simulink model "simerr"  (Simulink 7.3)
settings: Solver=ode45  StartTime=0.0  StopTime=10.0  RelTol=1e-3
values from neighbouring files (symbols this model uses):
  c = v(1:D)    [canon_proj.m]
undefined symbols (not defined in the file or in its folder): a, bth, by
settings Model: Creator=locomotion  LastModifiedBy=locomotion

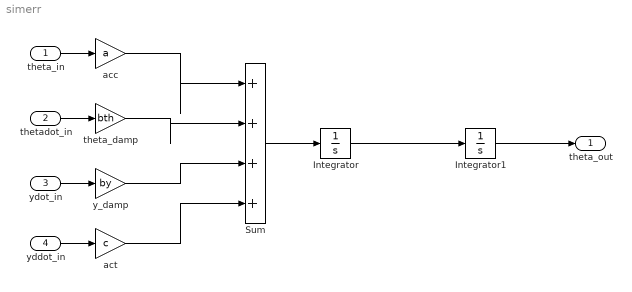
== system simerr ==
  theta_in : Inport  OutDataType=fixdt(1, 16)  OutScaling=2^0
  thetadot_in : Inport  Port=2  OutDataType=fixdt(1, 16)  OutScaling=2^0
  ydot_in : Inport  Port=3  OutDataType=fixdt(1, 16)  OutScaling=2^0
  yddot_in : Inport  Port=4  OutDataType=fixdt(1, 16)  OutScaling=2^0
  Integrator : Integrator
  Integrator1 : Integrator
  Sum : Sum  Inputs=|++++  OutDataType=fixdt(1, 16)  OutScaling=2^0
  acc : Gain  Gain=a  ParameterDataType=fixdt(1, 16)  ParameterScaling=2^0  OutDataType=fixdt(1, 16)  OutScaling=2^0
  act : Gain  Gain=c  ParameterDataType=fixdt(1, 16)  ParameterScaling=2^0  OutDataType=fixdt(1, 16)  OutScaling=2^0
  theta_damp : Gain  Gain=bth  ParameterDataType=fixdt(1, 16)  ParameterScaling=2^0  OutDataType=fixdt(1, 16)  OutScaling=2^0
  y_damp : Gain  Gain=by  ParameterDataType=fixdt(1, 16)  ParameterScaling=2^0  OutDataType=fixdt(1, 16)  OutScaling=2^0
  theta_out : Outport  OutDataType=fixdt(1, 16)  OutScaling=2^0
  wires:
  theta_in/1 -> acc/1
  thetadot_in/1 -> theta_damp/1
  ydot_in/1 -> y_damp/1
  yddot_in/1 -> act/1
  acc/1 -> Sum/1
  theta_damp/1 -> Sum/2
  y_damp/1 -> Sum/3
  act/1 -> Sum/4
  Sum/1 -> Integrator/1
  Integrator/1 -> Integrator1/1
  Integrator1/1 -> theta_out/1
